simulink model "IFS_Sim"  (R2024b)
settings: Solver=ode23t  StartTime=0  StopTime=Sch_Cycle(end,1)  RelTol=1e-3
InitFcn:
  | IFS_Sim_Vehicle_Params
values from neighbouring files (symbols this model uses):
  Battery_Capacity = 8.5    [IFS_Sim_Vehicle_Params.m]
  Battery_Initial_SOC = 0.9    [IFS_Sim_Vehicle_Params.m]
  Battery_Voltage = n_series*n_stacks*max_cellV    (= 399)    [IFS_Sim_Vehicle_Params.m]
  MGA_Max_Torque = 240    [IFS_Sim_Vehicle_Params.m]
  Ts = 1    [IFS_Sim_Vehicle_Params.m]
libraries: nesl_utility x9, fl_lib x6, sdl_lib x3, slpidlib x1
settings Model: Creator=raulmoran  LastModifiedBy=raulmoran
settings DataIOCC: SaveFormat=StructureWithTime
settings OptimizationCC: BlockReduction=off  BufferReuse=off
settings DebuggingCC: AlgebraicLoopMsg=none
settings ExplorerConfigSet: SimMechanicsOpenEditorOnUpdate=off

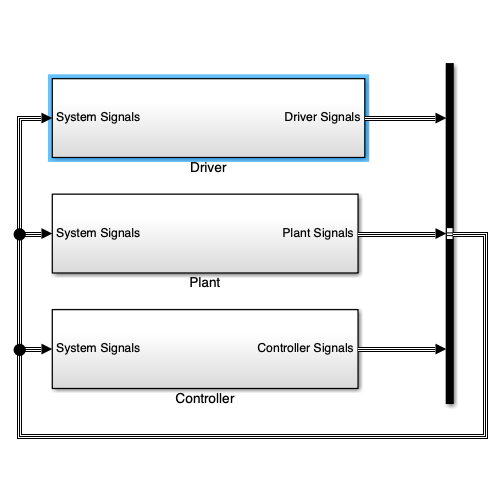
[thumbnail: Simulink's stored preview of the top-level diagram]
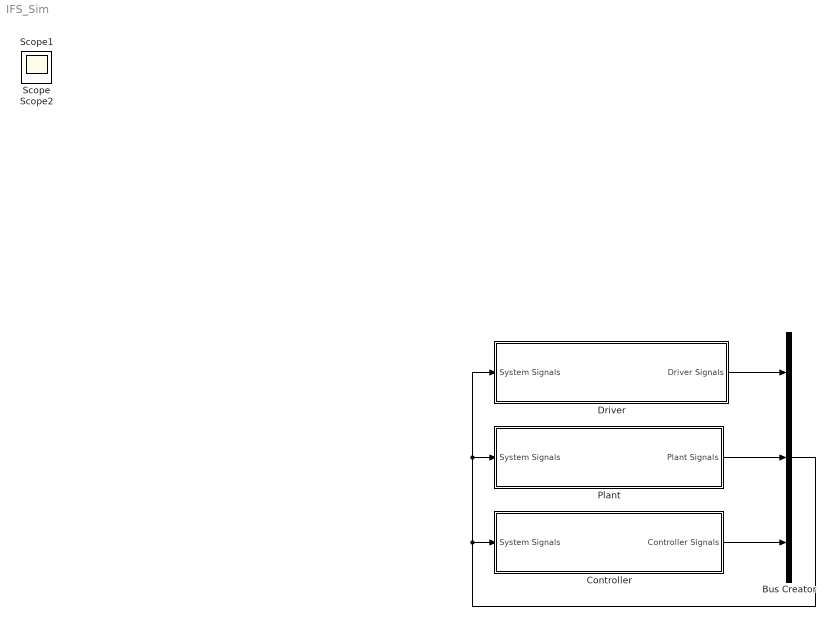
== system IFS_Sim ==
  Bus Creator : BusCreator  Inputs=3
  Controller : Subsystem
  Driver : Subsystem
  Plant : Subsystem
  Scope : Scope
  Scope1 : Scope
  Scope2 : Scope
  wires:
  Plant/1(Plant Signals) -> Bus Creator/2
  Driver/1(Driver Signals) -> Bus Creator/1
  Controller/1(Controller Signals) -> Bus Creator/3
  Bus Creator/1 -> Driver/1(System Signals), Plant/1(System Signals), Controller/1(System Signals)

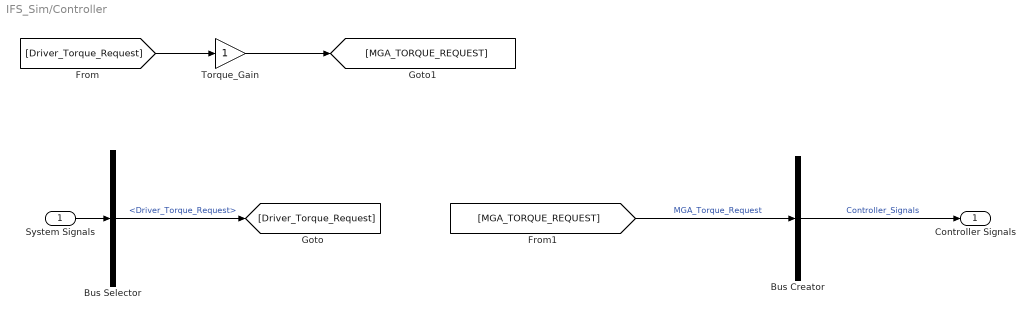
== system IFS_Sim/Controller ==
  System Signals : Inport
  Bus Creator : BusCreator  Inputs=1
  Bus Selector : BusSelector  OutputSignals=Driver_Signals.Driver_Torque_Request
  Torque_Gain : Gain
  Controller Signals : Outport
  wires:
  Bus Creator/1 -> Controller Signals/1  "Controller_Signals"
  System Signals/1 -> Bus Selector/1
  [MGA_TORQUE_REQUEST] -> Bus Creator/1  "MGA_Torque_Request"
  Bus Selector/1 -> [Driver_Torque_Request]  "<Driver_Torque_Request>"
  [Driver_Torque_Request] -> Torque_Gain/1
  Torque_Gain/1 -> [MGA_TORQUE_REQUEST]

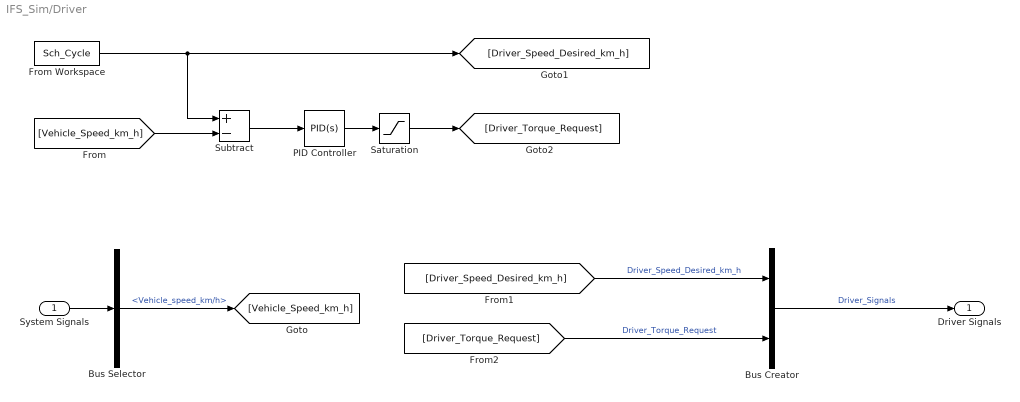
== system IFS_Sim/Driver ==
  System Signals : Inport
  Bus Creator : BusCreator  Inputs=2
  Bus Selector : BusSelector  OutputSignals=Plant_Signals.Vehicle_Signals.Vehicle_speed_km/h
  From Workspace : FromWorkspace  VariableName=Sch_Cycle
  PID Controller : slpidlib/PID Controller  Controller=PID  Form=Parallel  TimeDomain=Continuous-time  UseExternalTs=off  SampleTime=-1  IntegratorMethod=Forward Euler  FilterMethod=Forward Euler  ControllerParametersSource=internal  P=0.208124609499335  I=0.192924953430325  UseKiTs=off  D=0.00753137617644429  UseExternalDerivativeSource=off  N=19.1388047645984  UseFilter=on  TunerSelectOption=Transfer Function Based (PID Tuner App)  InitialConditionSource=internal  InitialConditionForIntegrator=0  InitialConditionForFilter=0  DifferentiatorICPrevScaledInput=0  ExternalReset=none  TrackingMode=off  Kt=1  LimitOutput=off  SatLimitsSource=internal  UpperSaturationLimit=inf  LowerSaturationLimit=-inf  LinearizeAsGain=on  AntiWindupMode=none  Kb=1  LimitIntegrator=off  UpperIntegratorSaturationLimit=inf  LowerIntegratorSaturationLimit=-inf  POutMin=[]  POutMax=[]  IOutMin=[]  IOutMax=[]  DOutMin=[]  DOutMax=[]  NOutMin=[]  NOutMax=[]  SumOutMin=[]  SumOutMax=[]  SaturationOutMin=[]  SaturationOutMax=[]  PParamMin=[]  PParamMax=[]  IParamMin=[]  IParamMax=[]  DParamMin=[]  DParamMax=[]  NParamMin=[]  NParamMax=[]  KbParamMin=[]  KbParamMax=[]  KtParamMin=[]  KtParamMax=[]  KbOutMin=[]  KbOutMax=[]  KtOutMin=[]  KtOutMax=[]  IntegratorOutMin=[]  IntegratorOutMax=[]  FilterOutMin=[]  FilterOutMax=[]  SumI1OutMin=[]  SumI1OutMax=[]  SumI2OutMin=[]  SumI2OutMax=[]  SumI3OutMin=[]  SumI3OutMax=[]  SumI4OutMin=[]  SumI4OutMax=[]  SumDOutMin=[]  SumDOutMax=[]  DifferentiatorOutMin=[]  DifferentiatorOutMax=[]  FilterDiffOutCoefMin=[]  FilterDiffOutCoefMax=[]  ReciprocalOutMin=[]  ReciprocalOutMax=[]  SumDenOutMin=[]  SumDenOutMax=[]  SumNumOutMin=[]  SumNumOutMax=[]  DivideOutMin=[]  DivideOutMax=[]  UdiffTsProdOutMin=[]  UdiffTsProdOutMax=[]  NTsProdOutMin=[]  NTsProdOutMax=[]  UintegralTsProdOutMin=[]  UintegralTsProdOutMax=[]  UngainTsProdOutMin=[]  UngainTsProdOutMax=[]  ClampingZeroOutDataTypeStr=Inherit: Inherit via back propagation  ClampingZeroOutMin=[]  ClampingZeroOutMax=[]  FilterDenConstantOutDataTypeStr=Inherit: Inherit via back propagation  FilterDenConstantOutMin=[]  FilterDenConstantOutMax=[]  PCopyOutDataTypeStr=Inherit: Inherit via back propagation  PCopyOutMin=[]  PCopyOutMax=[]  NCopyOutDataTypeStr=Inherit: Inherit via back propagation  NCopyOutMin=[]  NCopyOutMax=[]  IntegratorContinuousStateAttributes=''  IntegratorStateMustResolveToSignalObject=off  IntegratorRTWStateStorageClass=Auto  FilterContinuousStateAttributes=''  FilterStateMustResolveToSignalObject=off  FilterRTWStateStorageClass=Auto  ParallelPVariant=InternalParameters  IdealPVariant=Disabled  IVariant=InternalParameters  DVariant=InternalParameters  IntegratorVariant=Continuous  SatVariant=Disabled  AWVariant=Passthrough  PCopyVariant=Disabled  TRVariant=Disabled  FdbkBlocksVariant=Forward  IdealPFdbkVariant=Disabled  SatFdbkVariant=Disabled  DerivativeFilterVariant=ContFilter  NVariant=InternalParameters  NCopyVariant=Disabled  FilterICVariant=InternalICsFilter  IntegratorICVariant=InternalICs  ExternalResetVariant=Disabled  TRSumVariant=Passthrough  SumFdbkVariant=Disabled  SumVariant=Sum_PID  TsampFilterVariant=InternalTs  TsampNgainVariant=Passthrough  TsampIntegralVariant=Disabled_SignalSpec  ExternalSaturationOutDataTypeStr=Inherit: Same as second input  DerivativeSourceVariant=ErrorSignal  PreIntVariant=InternalPreInt
  Saturation : Saturate  UpperLimit=1  LowerLimit=-1
  Subtract : Sum  Inputs=+-
  Driver Signals : Outport
  wires:
  System Signals/1 -> Bus Selector/1
  Bus Creator/1 -> Driver Signals/1  "Driver_Signals"
  [Driver_Torque_Request] -> Bus Creator/2  "Driver_Torque_Request"
  [Driver_Speed_Desired_km_h] -> Bus Creator/1  "Driver_Speed_Desired_km_h"
  Bus Selector/1 -> [Vehicle_Speed_km_h]  "<Vehicle_speed_km/h>"
  [Vehicle_Speed_km_h] -> Subtract/2
  Saturation/1 -> [Driver_Torque_Request]
  From Workspace/1 -> [Driver_Speed_Desired_km_h], Subtract/1
  PID Controller/1 -> Saturation/1
  Subtract/1 -> PID Controller/1

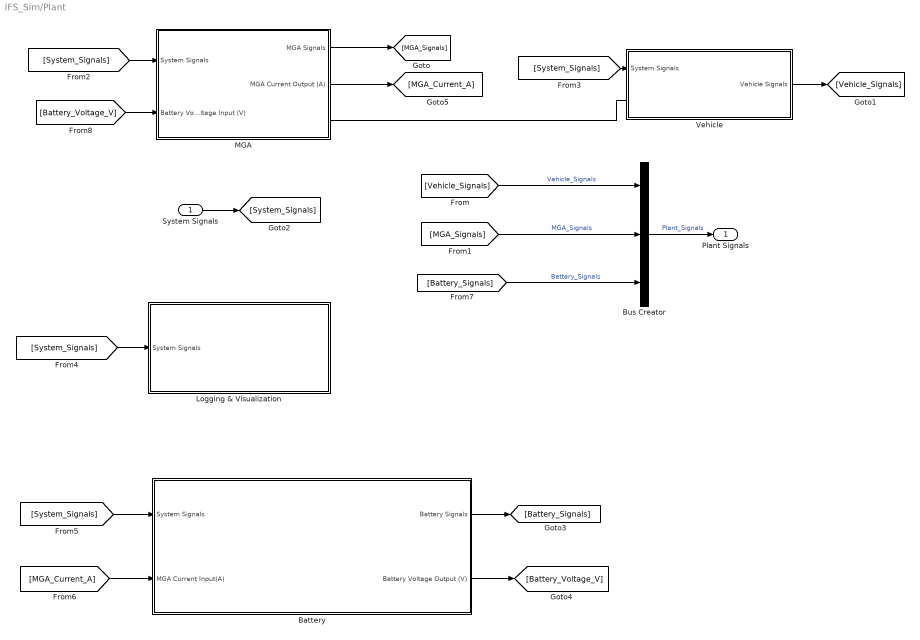
== system IFS_Sim/Plant ==
  System Signals : Inport
  Battery : Subsystem
  Bus Creator : BusCreator  Inputs=3
  Logging & Visualization : Subsystem
  MGA : Subsystem
  Vehicle : Subsystem
  Plant Signals : Outport
  wires:
  System Signals/1 -> [System_Signals]
  Bus Creator/1 -> Plant Signals/1  "Plant_Signals"
  [MGA_Signals] -> Bus Creator/2  "MGA_Signals"
  [Vehicle_Signals] -> Bus Creator/1  "Vehicle_Signals"
  MGA/1(MGA Signals) -> [MGA_Signals]
  Vehicle/1(Vehicle Signals) -> [Vehicle_Signals]
  [System_Signals] -> MGA/1(System Signals)
  [System_Signals] -> Vehicle/1(System Signals)
  [System_Signals] -> Logging & Visualization/1(System Signals)
  Battery/1(Battery Signals) -> [Battery_Signals]
  Battery/2(Battery Voltage Output (V)) -> [Battery_Voltage_V]
  [MGA_Current_A] -> Battery/2(MGA Current Input(A))
  [System_Signals] -> Battery/1(System Signals)
  [Battery_Signals] -> Bus Creator/3  "Battery_Signals"
  [Battery_Voltage_V] -> MGA/2(Battery Voltage Input (V))
  MGA/2(MGA Current Output (A)) -> [MGA_Current_A]
  connections:
  MGA/RConn1 -- Vehicle/LConn1

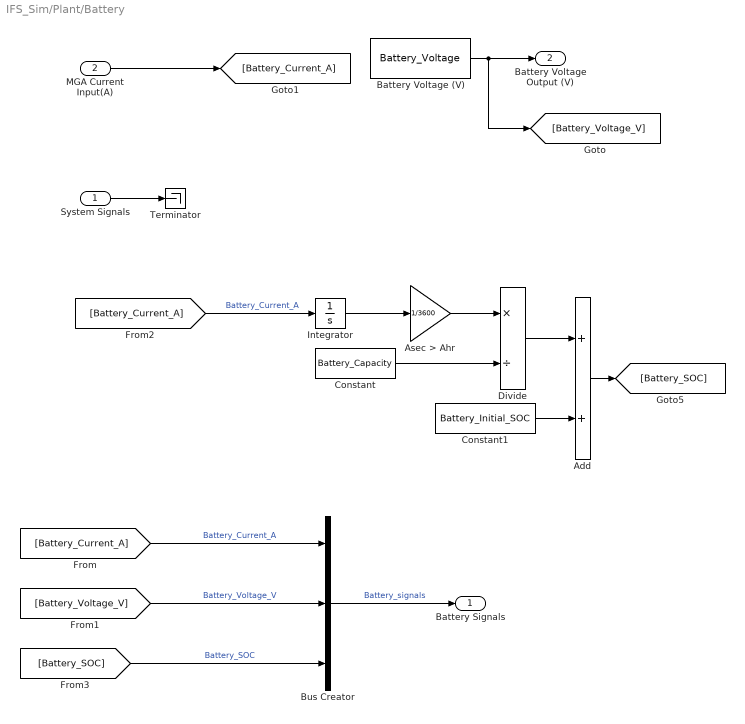
== system IFS_Sim/Plant/Battery ==
  System Signals : Inport
  MGA Current Input(A) : Inport  Port=2
  Add : Sum
  Asec > Ahr : Gain  Gain=1/3600
  Battery Voltage (V) : Constant  Value=Battery_Voltage
  Bus Creator : BusCreator  Inputs=3
  Constant : Constant  Value=Battery_Capacity
  Constant1 : Constant  Value=Battery_Initial_SOC
  Divide : Product  Inputs=*/
  Integrator : Integrator
  Terminator : Terminator
  Battery Signals : Outport
  Battery Voltage Output (V) : Outport  Port=2
  wires:
  Bus Creator/1 -> Battery Signals/1  "Battery_signals"
  [Battery_Current_A] -> Bus Creator/1  "Battery_Current_A"
  [Battery_Voltage_V] -> Bus Creator/2  "Battery_Voltage_V"
  System Signals/1 -> Terminator/1
  Battery Voltage (V)/1 -> [Battery_Voltage_V], Battery Voltage Output (V)/1
  MGA Current Input(A)/1 -> [Battery_Current_A]
  [Battery_Current_A] -> Integrator/1  "Battery_Current_A"
  Integrator/1 -> Asec > Ahr/1
  Asec > Ahr/1 -> Divide/1
  Constant/1 -> Divide/2
  Divide/1 -> Add/1
  Constant1/1 -> Add/2
  Add/1 -> [Battery_SOC]
  [Battery_SOC] -> Bus Creator/3  "Battery_SOC"

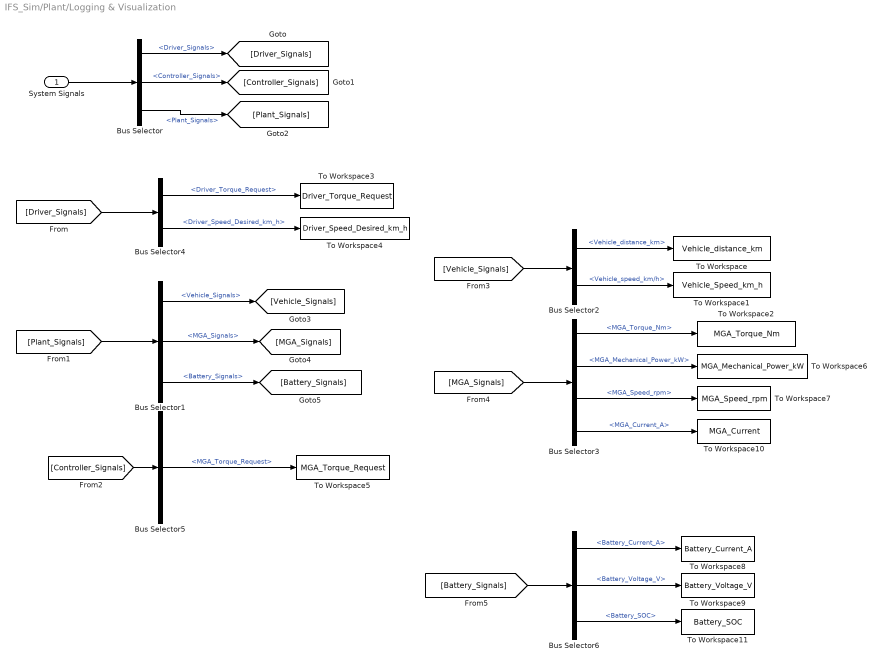
== system IFS_Sim/Plant/Logging & Visualization ==
  System Signals : Inport
  Bus Selector : BusSelector  OutputSignals=Driver_Signals,Controller_Signals,Plant_Signals
  Bus Selector1 : BusSelector  OutputSignals=Vehicle_Signals,MGA_Signals,Battery_Signals
  Bus Selector2 : BusSelector  OutputSignals=Vehicle_distance_km,Vehicle_speed_km/h
  Bus Selector3 : BusSelector  OutputSignals=MGA_Torque_Nm,MGA_Mechanical_Power_kW,MGA_Speed_rpm,MGA_Current_A
  Bus Selector4 : BusSelector  OutputSignals=Driver_Torque_Request,Driver_Speed_Desired_km_h
  Bus Selector5 : BusSelector  OutputSignals=MGA_Torque_Request
  Bus Selector6 : BusSelector  OutputSignals=Battery_Current_A,Battery_Voltage_V,Battery_SOC
  To Workspace : ToWorkspace  VariableName=Vehicle_distance_km  SampleTime=Ts
  To Workspace1 : ToWorkspace  VariableName=Vehicle_Speed_km_h  SampleTime=Ts
  To Workspace10 : ToWorkspace  VariableName=MGA_Current  SaveFormat=Timeseries  SampleTime=-1
  To Workspace11 : ToWorkspace  VariableName=Battery_SOC  SaveFormat=Timeseries  SampleTime=-1
  To Workspace2 : ToWorkspace  VariableName=MGA_Torque_Nm  SaveFormat=Timeseries  SampleTime=-1
  To Workspace3 : ToWorkspace  VariableName=Driver_Torque_Request  SaveFormat=Timeseries  SampleTime=-1
  To Workspace4 : ToWorkspace  VariableName=Driver_Speed_Desired_km_h  SaveFormat=Timeseries  SampleTime=-1
  To Workspace5 : ToWorkspace  VariableName=MGA_Torque_Request  SaveFormat=Timeseries  SampleTime=-1
  To Workspace6 : ToWorkspace  VariableName=MGA_Mechanical_Power_kW  SaveFormat=Timeseries  SampleTime=-1
  To Workspace7 : ToWorkspace  VariableName=MGA_Speed_rpm  SaveFormat=Timeseries  SampleTime=-1
  To Workspace8 : ToWorkspace  VariableName=Battery_Current_A  SaveFormat=Timeseries  SampleTime=-1
  To Workspace9 : ToWorkspace  VariableName=Battery_Voltage_V  SaveFormat=Timeseries  SampleTime=-1
  wires:
  System Signals/1 -> Bus Selector/1
  Bus Selector/1 -> [Driver_Signals]  "<Driver_Signals>"
  Bus Selector/2 -> [Controller_Signals]  "<Controller_Signals>"
  Bus Selector/3 -> [Plant_Signals]  "<Plant_Signals>"
  [Plant_Signals] -> Bus Selector1/1
  Bus Selector1/1 -> [Vehicle_Signals]  "<Vehicle_Signals>"
  Bus Selector1/2 -> [MGA_Signals]  "<MGA_Signals>"
  [Vehicle_Signals] -> Bus Selector2/1
  [MGA_Signals] -> Bus Selector3/1
  Bus Selector2/1 -> To Workspace/1  "<Vehicle_distance_km>"
  Bus Selector2/2 -> To Workspace1/1  "<Vehicle_speed_km/h>"
  Bus Selector3/1 -> To Workspace2/1  "<MGA_Torque_Nm>"
  [Driver_Signals] -> Bus Selector4/1
  Bus Selector4/1 -> To Workspace3/1  "<Driver_Torque_Request>"
  Bus Selector4/2 -> To Workspace4/1  "<Driver_Speed_Desired_km_h>"
  [Controller_Signals] -> Bus Selector5/1
  Bus Selector5/1 -> To Workspace5/1  "<MGA_Torque_Request>"
  Bus Selector3/2 -> To Workspace6/1  "<MGA_Mechanical_Power_kW>"
  Bus Selector3/3 -> To Workspace7/1  "<MGA_Speed_rpm>"
  Bus Selector1/3 -> [Battery_Signals]  "<Battery_Signals>"
  [Battery_Signals] -> Bus Selector6/1
  Bus Selector6/1 -> To Workspace8/1  "<Battery_Current_A>"
  Bus Selector6/2 -> To Workspace9/1  "<Battery_Voltage_V>"
  Bus Selector3/4 -> To Workspace10/1  "<MGA_Current_A>"
  Bus Selector6/3 -> To Workspace11/1  "<Battery_SOC>"

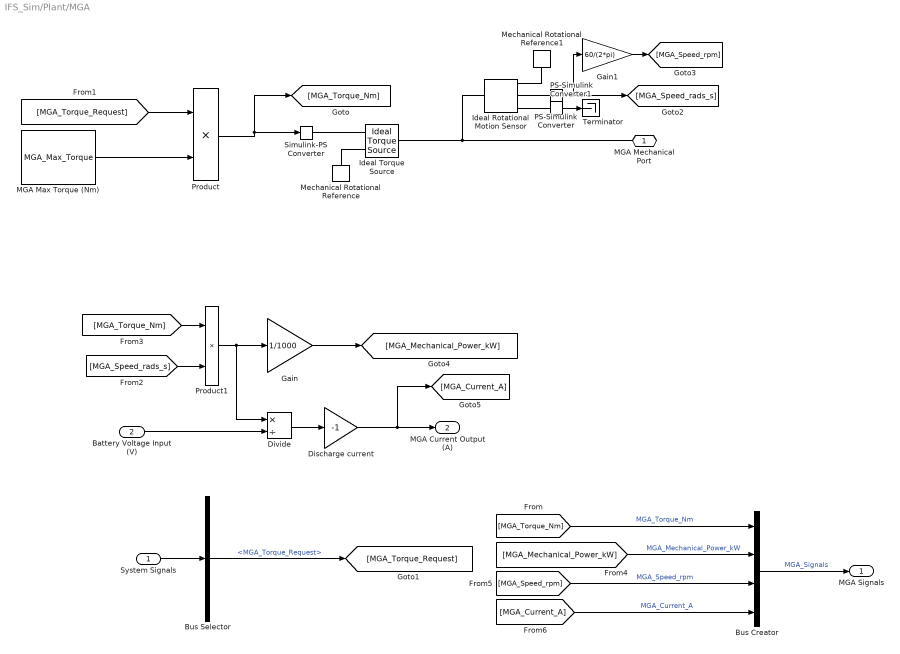
== system IFS_Sim/Plant/MGA ==
  System Signals : Inport
  Battery Voltage Input (V) : Inport  Port=2
  Bus Creator : BusCreator  Inputs=4
  Bus Selector : BusSelector  OutputSignals=Controller_Signals.MGA_Torque_Request
  Discharge current : Gain  Gain=-1
  Divide : Product  Inputs=*/
  Gain : Gain  Gain=1/1000
  Gain1 : Gain  Gain=60/(2*pi)
  Ideal Rotational Motion Sensor : fl_lib/Mechanical/Mechanical Sensors/Ideal Rotational Motion Sensor  reference=foundation.enum.MeasurementReference.difference  acceleration_port=false  velocity_port=true  position_port=true  wrap_angle=false  offset=0 rad
  Ideal Torque Source : fl_lib/Mechanical/Mechanical Sources/Ideal Torque Source
  MGA Max Torque (Nm) : Constant  Value=MGA_Max_Torque
  Mechanical Rotational Reference : fl_lib/Mechanical/Rotational Elements/Mechanical Rotational Reference
  Mechanical Rotational Reference1 : fl_lib/Mechanical/Rotational Elements/Mechanical Rotational Reference
  PS-Simulink Converter : nesl_utility/PS-Simulink Converter  PhysicalDomain=network_engine_domain  SubClassName=ps_output  LeftPortType=input  RightPortType=output  PseudoPeriodic=off  Frequencies=[]  VectorFormat=inherit  Unit=inherit  AffineConversion=off
  PS-Simulink Converter1 : nesl_utility/PS-Simulink Converter  PhysicalDomain=network_engine_domain  SubClassName=ps_output  LeftPortType=input  RightPortType=output  PseudoPeriodic=off  Frequencies=[]  VectorFormat=inherit  Unit=inherit  AffineConversion=off
  Product : Product
  Product1 : Product
  Simulink-PS Converter : nesl_utility/Simulink-PS Converter  PhysicalDomain=network_engine_domain  SubClassName=ps_input  LeftPortType=input  RightPortType=output  PseudoPeriodic=off  Frequencies=[]  NoiseDistribution=none  NoiseParameters=[]  Unit=1  AffineConversion=off  FilteringAndDerivatives=provide  SimscapeFilterOrder=1  InputFilterTimeConstant=0.001  UdotUserProvided=0
  Terminator : Terminator
  MGA Mechanical Port : PMIOPort  Side=Right
  MGA Signals : Outport
  MGA Current Output (A) : Outport  Port=2
  wires:
  Bus Creator/1 -> MGA Signals/1  "MGA_Signals"
  System Signals/1 -> Bus Selector/1
  [MGA_Torque_Nm] -> Bus Creator/1  "MGA_Torque_Nm"
  Bus Selector/1 -> [MGA_Torque_Request]  "<MGA_Torque_Request>"
  MGA Max Torque (Nm)/1 -> Product/2
  Product/1 -> [MGA_Torque_Nm], Simulink-PS Converter/1
  [MGA_Torque_Request] -> Product/1
  PS-Simulink Converter1/1 -> Terminator/1
  PS-Simulink Converter/1 -> Gain1/1, [MGA_Speed_rads_s]
  Gain1/1 -> [MGA_Speed_rpm]
  Product1/1 -> Divide/1, Gain/1
  [MGA_Speed_rads_s] -> Product1/2
  [MGA_Torque_Nm] -> Product1/1
  Gain/1 -> [MGA_Mechanical_Power_kW]
  [MGA_Mechanical_Power_kW] -> Bus Creator/2  "MGA_Mechanical_Power_kW"
  [MGA_Speed_rpm] -> Bus Creator/3  "MGA_Speed_rpm"
  Battery Voltage Input (V)/1 -> Divide/2
  Divide/1 -> Discharge current/1
  Discharge current/1 -> [MGA_Current_A], MGA Current Output (A)/1
  [MGA_Current_A] -> Bus Creator/4  "MGA_Current_A"
  connections:
  Ideal Torque Source/RConn1 -- Simulink-PS Converter/RConn1
  MGA Mechanical Port/RConn1 -- Ideal Rotational Motion Sensor/LConn1 -- Ideal Torque Source/LConn1
  Mechanical Rotational Reference/LConn1 -- Ideal Torque Source/RConn2
  Ideal Rotational Motion Sensor/RConn1 -- Mechanical Rotational Reference1/LConn1
  Ideal Rotational Motion Sensor/RConn3 -- PS-Simulink Converter1/LConn1
  PS-Simulink Converter/LConn1 -- Ideal Rotational Motion Sensor/RConn2

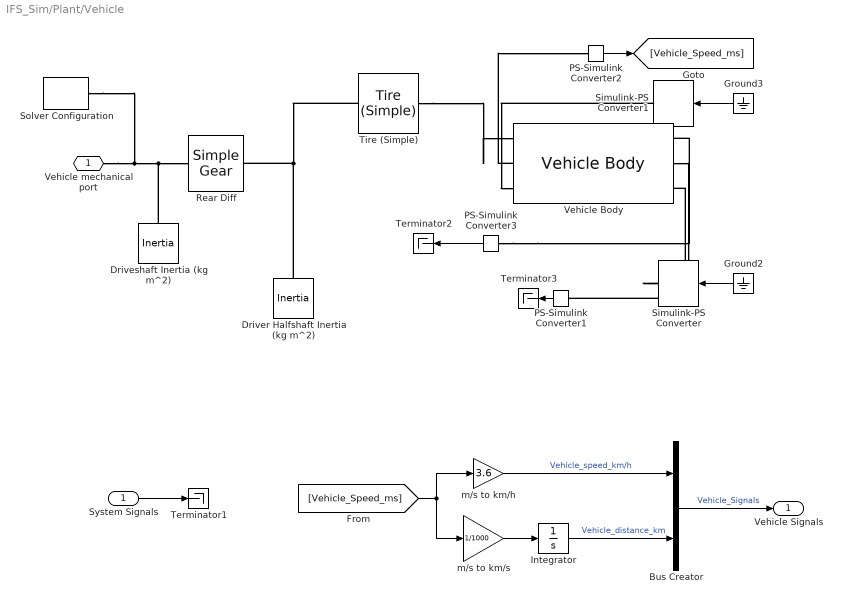
== system IFS_Sim/Plant/Vehicle ==
  System Signals : Inport
  Bus Creator : BusCreator  Inputs=2
  Driver Halfshaft Inertia (kg m^2) : fl_lib/Mechanical/Rotational Elements/Inertia  inertia=Vehicle_Dr_Shaft_Inertia kg*m^2  num_ports=foundation.enum.numPorts2.one  w_specify=off  w_priority=High  w=0 rad/s  w_nominal_specify=off  w_nominal_value=1  w_nominal_unit=rad/s  t_specify=off  t_priority=None  t=0 N*m  t_nominal_specify=off  t_nominal_value=1  t_nominal_unit=N*m
  Driveshaft Inertia (kg m^2) : fl_lib/Mechanical/Rotational Elements/Inertia  inertia=Vehicle_DShaft_Inertia kg*m^2  num_ports=foundation.enum.numPorts2.one  w_specify=off  w_priority=High  w=0 rad/s  w_nominal_specify=off  w_nominal_value=1  w_nominal_unit=rad/s  t_specify=off  t_priority=None  t=0 N*m  t_nominal_specify=off  t_nominal_value=1  t_nominal_unit=N*m
  Ground2 : Ground
  Ground3 : Ground
  Integrator : Integrator
  PS-Simulink Converter1 : nesl_utility/PS-Simulink Converter  PhysicalDomain=network_engine_domain  SubClassName=ps_output  LeftPortType=input  RightPortType=output  PseudoPeriodic=off  Frequencies=[]  VectorFormat=inherit  Unit=inherit  AffineConversion=off
  PS-Simulink Converter2 : nesl_utility/PS-Simulink Converter  PhysicalDomain=network_engine_domain  SubClassName=ps_output  LeftPortType=input  RightPortType=output  PseudoPeriodic=off  Frequencies=[]  VectorFormat=inherit  Unit=inherit  AffineConversion=off
  PS-Simulink Converter3 : nesl_utility/PS-Simulink Converter  PhysicalDomain=network_engine_domain  SubClassName=ps_output  LeftPortType=input  RightPortType=output  PseudoPeriodic=off  Frequencies=[]  VectorFormat=inherit  Unit=inherit  AffineConversion=off
  Rear Diff : sdl_lib/Gears/Simple Gear  ratio=Vehicle_Rear_Diff_Ratio  rotation_direction=sdl.enum.shaftOutputDirection.same  friction_model=sdl.enum.gear_efficiencies_load.off  T_noload=0.1 N*m  T_nom=5 N*m  efficiency_nom=0.8  efficiency=0.8  temperature_TLU=[280, 300, 320] K  load_TLU=[1, 5, 10] N*m  efficiency_TLU=[.95, .9, .85]  efficiency_TLU2=[.85, .8, .75; .95, .9, .85; .85, .8, .7]  w_thr=0.01 rad/s  pwr_thr=0.001 W  enable_backlash=false  hardstop_model=simscape.enum.hardstop.smooth  backlash_distance=1e-3 mm  r_base=0.1 m  transition=1e-4 mm  backlash_stiffness=1e6 N/m  backlash_damping=1e3 N*s/m  coeff_rest=0.7  v_tol=0.001 m/s  f_tol=0.001 N  mu_visc=[0, 0] N*m*s/rad  thermal_mass=50 J/K  temperature_specify=off  temperature_priority=High  temperature=300 K  temperature_nominal_specify=off  temperature_nominal_value=1  temperature_nominal_unit=K  x_backlash_specify=off  x_backlash_priority=None  x_backlash=0 mm  x_backlash_nominal_specify=off  x_backlash_nominal_value=1  x_backlash_nominal_unit=mm  f_hardstop_specify=off  f_hardstop_priority=None  f_hardstop=0 N  f_hardstop_nominal_specify=off  f_hardstop_nominal_value=1  f_hardstop_nominal_unit=N  v_backlash_specify=off  v_backlash_priority=None  v_backlash=0 m/s  v_backlash_nominal_specify=off  v_backlash_nominal_value=1  v_backlash_nominal_unit=m/s
  Simulink-PS Converter : nesl_utility/Simulink-PS Converter  PhysicalDomain=network_engine_domain  SubClassName=ps_input  LeftPortType=input  RightPortType=output  PseudoPeriodic=off  Frequencies=[]  NoiseDistribution=none  NoiseParameters=[]  Unit=1  AffineConversion=off  FilteringAndDerivatives=provide  SimscapeFilterOrder=1  InputFilterTimeConstant=0.001  UdotUserProvided=0
  Simulink-PS Converter1 : nesl_utility/Simulink-PS Converter  PhysicalDomain=network_engine_domain  SubClassName=ps_input  LeftPortType=input  RightPortType=output  PseudoPeriodic=off  Frequencies=[]  NoiseDistribution=none  NoiseParameters=[]  Unit=1  AffineConversion=off  FilteringAndDerivatives=provide  SimscapeFilterOrder=1  InputFilterTimeConstant=0.001  UdotUserProvided=0
  Solver Configuration : nesl_utility/Solver Configuration  PhysicalDomain=network_engine_domain  SubClassName=solver  LeftPortType=input  RightPortType=generic  Tones=[]  Harmonics=[]  SimulateNoise=off  Profile=off  UseLocalSampling=off  EnableSwitchedLinearOptims=on  FrequencyDomain=off  UseCCode=off  RelTol=0.001  AbsTol=0.001  MinStep=1e-09  ToWorkspace=off  RevertToSquareIcSolve=off  NumHomotopyIterations=100  PhasorMode=off  PhasorModeNumHarmonics=1  ConsistencySolver=NEWTON_XTOL_AFTER_FTOL  IndexReductionMethod=DerivativeReplacement  DoDC=off  ResidualTolerance=1e-09  ConsistencyTolSource=GLOBAL  ConsistencyAbsTol=0.001  ConsistencyRelTol=0.001  ConsistencyTolFactor=0.001  UseLocalSolver=off  LocalSolverChoice=NE_BACKWARD_EULER_ADVANCER  ResolveIndetEquations=on  FunctionEvalNumThread=1  LocalSolverSampleTime=0.001  DoFixedCost=off  MaxNonlinIter=3  MaxModeIter=2  ComputeImpulses=off  ImpulseIterations=2  LinearAlgebra=auto  LinearAlgebraNumThread=0  EquationFormulation=NE_TIME_EF  DelaysMemoryBudget=1024  AutomaticFiltering=on  FilteringTimeConstant=0.001  PartitionStorageMethod=AS_NEEDED  PartitionMemoryBudget=1024  PartitionMethod=ROBUST  MultibodyUseLocalSolver=off  MultibodyLocalSolverChoice=ODE1  MultibodyLocalSolverSampleTime=0.001
  Terminator1 : Terminator
  Terminator2 : Terminator
  Terminator3 : Terminator
  Tire (Simple) : sdl_lib/Tires & Vehicles/Tire (Simple)  r_tire=0.3 m  model_compliance=sdl.enum.compliance.off  stiffness=1e6 N/m  damping=1000 N*s/m  model_inertia=sdl.enum.model_inertia.on  tire_inertia=Wheel_Plus_Tire_Inertia kg*m^2  initial_velocity=0 rad/s
      settings: InternalSimscapePortConfiguration="{\"Bottom\":[],\"Left\":[{\"id\":\"A\",\"label\":\"A\",\"type\":\"foundation.mechanical.rotational.rotational\"}],\"Right\":[{\"id\":\"H\",\"label\":\"H\",\"type\":\"foundation.mechanical.translational.translational\"}],\"Top\":[]}"
  Vehicle Body : sdl_lib/Tires & Vehicles/Vehicle Body  mass=Vehicle_Mass kg  n_w=2  x_f=1.4 m  x_r=1.6 m  y_c=0.5 m  mass_var=false  g=9.81 m/s^2  liftoff_warning=false  area=3 m^2  Cd_var=false  Cd=0.4  rho=1.18 kg/m^3  model_pitch=false  inertia=4000 kg*m^2  suspension_model=sdl.enum.linearTLU.linear  k_f=1e4 N/m  b_f=1e4 N*s/m  k_r=1e4 N/m  b_r=1e4 N*s/m  k_f_TLU=[-2000, -1000, 0, 1000, 2000] N  x_f_TLU=[-.4, -.2, 0, .2, .4] m  b_f_TLU=[-200, -100, 0, 100, 200] N  v_f_TLU=[-4, -2, 0, 2, 4] m/s  k_r_TLU=[-2000, -1000, 0, 1000, 2000] N  x_r_TLU=[-.4, -.2, 0, .2, .4] m  b_r_TLU=[-200, -100, 0, 100, 200] N  v_r_TLU=[-4, -2, 0, 2, 4] m/s  interp_method=simscape.enum.interpolation.linear  extrap_method=simscape.enum.extrapolation.linear  model_hardstop=false  upper_bound_f=.25 m  lower_bound_f=-.25 m  stop_k_f=1e6 N/m  stop_b_f=150 N*s/m  upper_bound_r=.25 m  lower_bound_r=-.25 m  stop_k_r=1e6 N/m  stop_b_r=150 N*s/m  initial_pitch=0 rad  initial_pitch_rate=0 rad/s  v_specify=off  v_priority=High  v=0 m/s  v_nominal_specify=off  v_nominal_value=1  v_nominal_unit=m/s
      settings: InternalSimscapePortConfiguration="{\"Bottom\":[{\"id\":\"NR\",\"label\":\"NR\",\"type\":\"output\"},{\"id\":\"NF\",\"label\":\"NF\",\"type\":\"output\"},{\"id\":\"beta\",\"label\":\"beta\",\"type\":\"input\"}],\"Left\":[{\"id\":\"H\",\"label\":\"H\",\"type\":\"foundation.mechanical.translational.translational\"}],\"Right\":[],\"Top\":[{\"id\":\"V\",\"label\":\"V\",\"type\":\"output\"},{\"id\":\"wind\",\"label\":\"W\",\"type\":\"input\"}]}"
  m/s to km/h : Gain  Gain=3.6
  m/s to km/s : Gain  Gain=1/1000
  Vehicle mechanical port : PMIOPort  Side=Left
  Vehicle Signals : Outport
  wires:
  Bus Creator/1 -> Vehicle Signals/1  "Vehicle_Signals"
  System Signals/1 -> Terminator1/1
  m/s to km/h/1 -> Bus Creator/1  "Vehicle_speed_km/h"
  Ground2/1 -> Simulink-PS Converter/1
  Ground3/1 -> Simulink-PS Converter1/1
  PS-Simulink Converter1/1 -> Terminator3/1
  PS-Simulink Converter2/1 -> [Vehicle_Speed_ms]
  [Vehicle_Speed_ms] -> m/s to km/h/1, m/s to km/s/1
  Integrator/1 -> Bus Creator/2  "Vehicle_distance_km"
  m/s to km/s/1 -> Integrator/1
  PS-Simulink Converter3/1 -> Terminator2/1
  connections:
  Vehicle mechanical port/RConn1 -- Solver Configuration/RConn1 -- Driveshaft Inertia (kg m^2)/LConn1 -- Rear Diff/LConn1
  Driver Halfshaft Inertia (kg m^2)/LConn1 -- Tire (Simple)/LConn1 -- Rear Diff/RConn1
  Simulink-PS Converter/RConn1 -- Vehicle Body/RConn3
  Simulink-PS Converter1/RConn1 -- Vehicle Body/LConn3
  Tire (Simple)/RConn1 -- Vehicle Body/LConn1
  Vehicle Body/RConn2 -- PS-Simulink Converter1/LConn1
  Vehicle Body/LConn2 -- PS-Simulink Converter2/LConn1
  PS-Simulink Converter3/LConn1 -- Vehicle Body/RConn1
